simulink library "UDPLib"  (R2016a)
settings: Solver=ode45  StartTime=0.0  StopTime=10.0  RelTol=1e-3
libraries: dspnetwork x2
settings Model: Creator=sannem  LastModifiedBy=sannem
settings DataIOCC: LimitDataPoints=on
settings DebuggingCC: AllowSymbolicDim=off

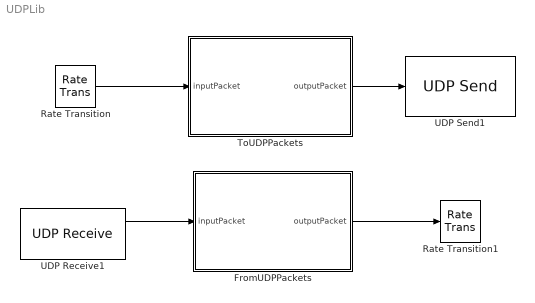
== system UDPLib ==
  FromUDPPackets : MATLAB Function  TreatAsAtomicUnit=on  mask{fullPacketSize=7200, bytesPerPacket=10000}
      mask prompts: fullPacketSize "Full packet size"; bytesPerPacket "Bytes per packet"
  Rate Transition : RateTransition  OutPortSampleTime=1/200
  Rate Transition1 : RateTransition  OutPortSampleTime=1/25
  ToUDPPackets : MATLAB Function  TreatAsAtomicUnit=on  mask{bytesPerPacket=10000}
      mask prompts: bytesPerPacket "Bytes per packet"
  UDP Receive1 : dspnetwork/UDP Receive  localURL='0.0.0.0'  localPort=24000  remoteURL='192.168.1.1'  remotePort=-1  recvBufferSize=73728  dims=15000  signalDatatype=uint8  isVarSize=off  showBlockingTime=off  blockingTime=0  sampletime=1/200
  UDP Send1 : dspnetwork/UDP Send
  wires:
  FromUDPPackets/1(outputPacket) -> Rate Transition1/1
  Rate Transition/1 -> ToUDPPackets/1(inputPacket)
  ToUDPPackets/1(outputPacket) -> UDP Send1/1
  UDP Receive1/1 -> FromUDPPackets/1(inputPacket)

== matlab function UDPLib/FromUDPPackets ==
  data: inputPacket input; bytesPerPacket parameter; outputPacket output; fullPacketSize parameter
function outputPacket  = FromUDPPackets(inputPacket, bytesPerPacket, fullPacketSize)

persistent tempOutputPacket     % packet where the incoming subpackets are written to
if isempty(tempOutputPacket)
    tempOutputPacket = zeros(1,fullPacketSize);
end

dataPerPacket = bytesPerPacket - 1; % remove 1 byte for the header  

header = double(inputPacket(1));
startIndex = 1;
if header > 0
    startIndex = ((header - 1) * dataPerPacket) + 1;
end
endIndex = min(header * dataPerPacket, fullPacketSize);
tempOutputPacket(startIndex : endIndex) = uint8(inputPacket(2 : endIndex - startIndex + 2));
outputPacket = uint8(tempOutputPacket);
% outputPacket = uint8(zeros(1,fullPacketSize));

end

== matlab function UDPLib/ToUDPPackets ==
  data: inputPacket input; outputPacket output; bytesPerPacket parameter
function outputPacket = ToUDPPackets(inputPacket, bytesPerPacket)

dataPerPacket = bytesPerPacket - 1; % remove 1 byte for the header

persistent counter  % keeps track of how many sub packets have been send
if isempty(counter)
   counter = 1;
end

persistent packetInBuffer % storage of the whole packet to be send
if isempty(packetInBuffer)
    packetInBuffer = inputPacket;
end

subPacketCount = length(inputPacket) / dataPerPacket;   % compute how many packets are needed
if (floor(subPacketCount) ~= subPacketCount || subPacketCount == 0 )  
   subPacketCount = floor(subPacketCount) + 1;  % Make sure the packet count is a whole number > 0
end

packetLength = dataPerPacket;
if (counter * dataPerPacket > length(packetInBuffer)) % if the sub packet is smaller than bitsPerPacket, adjust the packet length
    packetLength = mod(length(packetInBuffer),dataPerPacket); 
end

startIndex = dataPerPacket * (counter - 1) + 1;
outputPacket = uint8(zeros(1, bytesPerPacket));
outputPacket(1,1) = uint8(counter);  % add a header
outputPacket(1, 2 : packetLength + 1) =  uint8(inputPacket(startIndex : startIndex + packetLength ));

counter = counter + 1;
if counter > subPacketCount
   counter = 1;
   packetInBuffer = inputPacket; %  Put a new input packet in the buffer
end

end
